simulink library "librarySimulink"  (R2020b)
settings: Solver=VariableStepAuto  StartTime=0.0  StopTime=10.0  RelTol=1e-3
values from neighbouring files (symbols this model uses):
  MU = 398600    [linearControlTuning.m]
  n = sqrt(MU/a^3)    [linearControlTuning.m]
undefined symbols (not defined in the file or in its folder): A0, areaValues, gravityGradient, MAGNETIC_FIELD_INCLINATION, magneticTorque, N_EARTH, normalVects, nSurfaces, OBLIQUITY, orbit, positions, R_EARTH, rhoDValues, rhoSValues, spacecraft, SRP
libraries: $bdroot x34
settings Model: Creator=pacif  LastModifiedBy=pacif

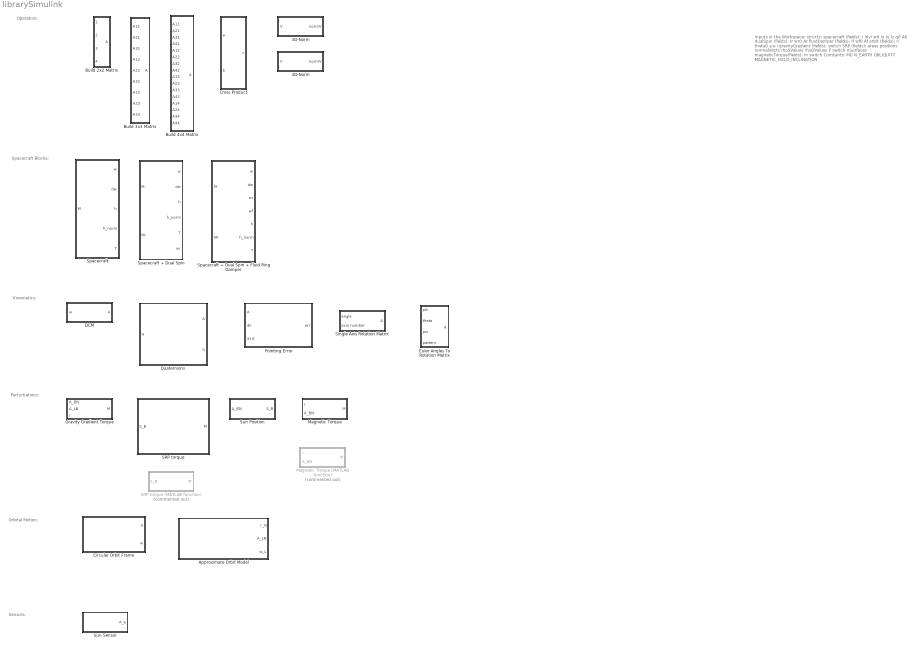
== system librarySimulink ==
  note: Operators:
  note: Inputs in the Workspace:
      |
      | structs:
      | spacecraft (fields):
      | I
      | invI
      | w0
      | Ix
      | Iy
      | Iz
      | q0
      | A0
      |
      | dualSpin (fields):
      | Ir
      | wr0
      | Ar
      | fluidDamper (fields):
      | If
      | wf0
      | Af
      | orbit (fields):
      | n
      | theta0
      | a
      | e
      | i
      | gravityGradient (fields):
      | switch
      | SRP (fields):
      | areas
      | positions
      | normalVects
      | rhoSValues
      | rhoDValues
      | P
      | switch
      | nSurfaces
      | magneticTorque(fields):
      | m
      | switch
      |
      | Constants:
      | MU
      | N_EARTH
      | OBLIQUITY
      | MAGNETIC_FIELD_INCLINATION
  note: Spacecraft Blocks:
  note: Kinematics:
  note: Perturbations:
  note: Orbital Motion:
  note: Sensors:
  3D-Norm : Subsystem
  4D-Norm : Subsystem
  Approximate Orbit Model : Subsystem
  Build 2x2 Matrix : Subsystem
  Build 3x3 Matrix : Subsystem
  Build 4x4 Matrix : Subsystem
  "Circular Orbit Frame " : Subsystem
  Cross Product : Subsystem
  DCM : Subsystem
  Euler Angles To Rotation Matrix : Subsystem
  Gravity Gradient Torque : Subsystem
  Magnetic Torque : Subsystem
  Magnetic Torque (MATLAB function) : Subsystem  Commented=on
  Pointing Error : Subsystem
  "Quaternions " : Subsystem
  SRP torque : Subsystem
  SRP torque (MATLAB function) : Subsystem  Commented=on
  Single Axis Rotation Matrix : Subsystem
  "Spacecraft " : Subsystem
  Spacecraft + Dual Spin : Subsystem  AncestorBlock=my_SADC_library/Spacecraft
  Spacecraft + Dual Spin + Fluid Ring Damper : Subsystem  AncestorBlock=my_SADC_library/Spacecraft
  "Sun Position " : Subsystem
  Sun Sensor : Subsystem

== system librarySimulink/3D-Norm ==
  V : Inport
  Add : Sum  Inputs=+++
  Demux : Demux  Outputs=3
  Square : Math  Operator=square  SaturateOnIntegerOverflow=on
  Square Root : Sqrt  SaturateOnIntegerOverflow=on
  Square1 : Math  Operator=square  SaturateOnIntegerOverflow=on
  Square2 : Math  Operator=square  SaturateOnIntegerOverflow=on
  normV : Outport
  wires:
  V/1 -> Demux/1
  Demux/3 -> Square2/1
  Demux/2 -> Square1/1
  Demux/1 -> Square/1
  Square/1 -> Add/1
  Square1/1 -> Add/2
  Square2/1 -> Add/3
  Add/1 -> Square Root/1
  Square Root/1 -> normV/1

== system librarySimulink/4D-Norm ==
  V : Inport
  Add : Sum  Inputs=++++
  Demux : Demux
  Square{,1..3} (4 alike) : Math  Operator=square  SaturateOnIntegerOverflow=on
  Square Root : Sqrt  SaturateOnIntegerOverflow=on
  normV : Outport
  wires:
  Square1/1 -> Add/2
  Demux/2 -> Square1/1
  V/1 -> Demux/1
  Demux/1 -> Square/1
  Square Root/1 -> normV/1
  Square2/1 -> Add/3
  Square/1 -> Add/1
  Demux/3 -> Square2/1
  Add/1 -> Square Root/1
  Demux/4 -> Square3/1
  Square3/1 -> Add/4

== system librarySimulink/Approximate Orbit Model ==
  Constant : Constant  Value=0
  Integrator : Integrator  InitialCondition=orbit.theta0
  Mux : Mux  Inputs=3
  Subsystem : Subsystem
  Subsystem1 : Subsystem
  Subsystem2 : Subsystem
  r_N : Outport
  A_LN : Outport  Port=2
  w_L : Outport  Port=3
  wires:
  Integrator/1 -> Subsystem2/1(theta), Subsystem1/1(theta), Subsystem/1(theta)
  Subsystem2/1(r_N) -> r_N/1
  Subsystem/1(theta_dot) -> Mux/3, Integrator/1
  Subsystem1/1(A_LN) -> A_LN/1
  Mux/1 -> w_L/1
  Constant/1 -> Mux/2, Mux/1

== system librarySimulink/Build 2x2 Matrix ==
  A11 : Inport
  A21 : Inport  Port=2
  A12 : Inport  Port=3
  A22 : Inport  Port=4
  Mux : Mux  Inputs=2
  Mux1 : Mux  Inputs=2
  Vector Concatenate : Concatenate  Mode=Multidimensional array  ConcatenateDimension=2
  A : Outport
  wires:
  Mux/1 -> Vector Concatenate/1
  Mux1/1 -> Vector Concatenate/2
  Vector Concatenate/1 -> A/1
  A11/1 -> Mux/1
  A22/1 -> Mux1/2
  A21/1 -> Mux/2
  A12/1 -> Mux1/1

== system librarySimulink/Build 3x3 Matrix ==
  A11 : Inport
  A21 : Inport  Port=2
  A31 : Inport  Port=3
  A12 : Inport  Port=4
  A22 : Inport  Port=5
  A32 : Inport  Port=6
  "A13 " : Inport  Port=7
  A23 : Inport  Port=8
  A33 : Inport  Port=9
  Mux : Mux  Inputs=3
  Mux1 : Mux  Inputs=3
  Mux2 : Mux  Inputs=3
  Vector Concatenate : Concatenate  NumInputs=3  Mode=Multidimensional array  ConcatenateDimension=2
  A : Outport
  wires:
  A11/1 -> Mux/1
  A21/1 -> Mux/2
  A31/1 -> Mux/3
  A12/1 -> Mux1/1
  A22/1 -> Mux1/2
  A32/1 -> Mux1/3
  "A13 "/1 -> Mux2/1
  A23/1 -> Mux2/2
  A33/1 -> Mux2/3
  Mux/1 -> Vector Concatenate/1
  Mux1/1 -> Vector Concatenate/2
  Mux2/1 -> Vector Concatenate/3
  Vector Concatenate/1 -> A/1

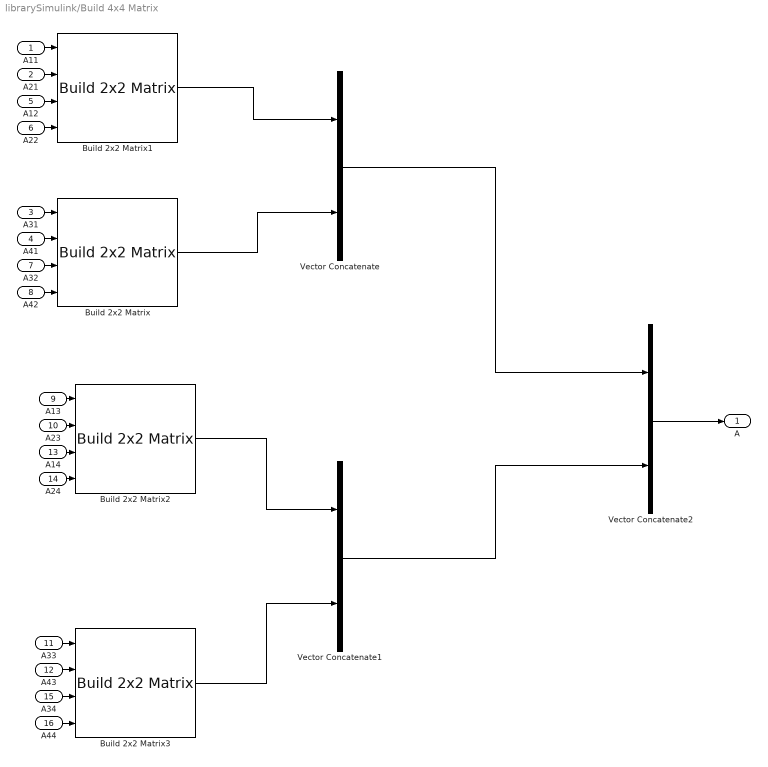
== system librarySimulink/Build 4x4 Matrix ==
  A11 : Inport
  A21 : Inport  Port=2
  A31 : Inport  Port=3
  A41 : Inport  Port=4
  A12 : Inport  Port=5
  A22 : Inport  Port=6
  A32 : Inport  Port=7
  A42 : Inport  Port=8
  A13 : Inport  Port=9
  A23 : Inport  Port=10
  A33 : Inport  Port=11
  A43 : Inport  Port=12
  A14 : Inport  Port=13
  A24 : Inport  Port=14
  A34 : Inport  Port=15
  A44 : Inport  Port=16
  Build 2x2 Matrix{,1..3} (4 alike) : $bdroot/Build 2x2 Matrix  SystemSampleTime=-1  VariantActivationTime=update diagram  Latency=0  AutoFrameSizeCalculation=off
  Vector Concatenate : Concatenate  Mode=Multidimensional array
  Vector Concatenate1 : Concatenate  Mode=Multidimensional array
  Vector Concatenate2 : Concatenate  Mode=Multidimensional array  ConcatenateDimension=2
  A : Outport
  wires:
  A11/1 -> Build 2x2 Matrix1/1
  A21/1 -> Build 2x2 Matrix1/2
  A12/1 -> Build 2x2 Matrix1/3
  A22/1 -> Build 2x2 Matrix1/4
  A13/1 -> Build 2x2 Matrix2/1
  A23/1 -> Build 2x2 Matrix2/2
  A14/1 -> Build 2x2 Matrix2/3
  A24/1 -> Build 2x2 Matrix2/4
  A31/1 -> Build 2x2 Matrix/1
  A41/1 -> Build 2x2 Matrix/2
  A32/1 -> Build 2x2 Matrix/3
  A42/1 -> Build 2x2 Matrix/4
  A33/1 -> Build 2x2 Matrix3/1
  A43/1 -> Build 2x2 Matrix3/2
  A34/1 -> Build 2x2 Matrix3/3
  A44/1 -> Build 2x2 Matrix3/4
  Build 2x2 Matrix1/1 -> Vector Concatenate/1
  Build 2x2 Matrix/1 -> Vector Concatenate/2
  Vector Concatenate/1 -> Vector Concatenate2/1
  Vector Concatenate1/1 -> Vector Concatenate2/2
  Vector Concatenate2/1 -> A/1
  Build 2x2 Matrix3/1 -> Vector Concatenate1/2
  Build 2x2 Matrix2/1 -> Vector Concatenate1/1

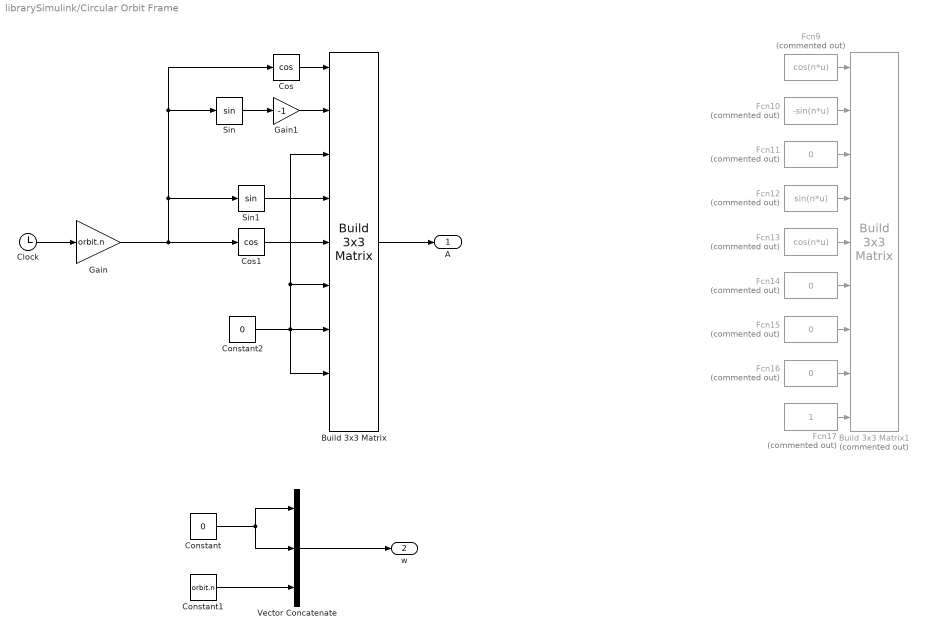
== system librarySimulink/Circular Orbit Frame  ==
  Build 3x3 Matrix : $bdroot/Build 3x3 Matrix  SystemSampleTime=-1  VariantActivationTime=update diagram  Latency=0  AutoFrameSizeCalculation=off
  Build 3x3 Matrix1 : $bdroot/Build 3x3 Matrix  Commented=on  SystemSampleTime=-1  VariantActivationTime=update diagram  Latency=0  AutoFrameSizeCalculation=off
  Clock : Clock
  Constant : Constant  Value=0
  Constant1 : Constant  Value=orbit.n
  Constant2 : Constant  Value=0
  Cos : Trigonometry  Operator=cos
  Cos1 : Trigonometry  Operator=cos
  Fcn10 : Fcn  Commented=on  Expr=-sin(n*u)
  Fcn{11,14..16} (4 alike) : Fcn  Commented=on  Expr=0
  Fcn12 : Fcn  Commented=on  Expr=sin(n*u)
  Fcn13 : Fcn  Commented=on  Expr=cos(n*u)
  Fcn17 : Fcn  Commented=on  Expr=1
  Fcn9 : Fcn  Commented=on  Expr=cos(n*u)
  Gain : Gain  Gain=orbit.n
  Gain1 : Gain  Gain=-1
  Sin : Trigonometry
  Sin1 : Trigonometry
  Vector Concatenate : Concatenate  NumInputs=3
  A : Outport
  w : Outport  Port=2
  wires:
  Cos/1 -> Build 3x3 Matrix/1
  Gain1/1 -> Build 3x3 Matrix/2
  Constant2/1 -> Build 3x3 Matrix/8, Build 3x3 Matrix/6, Build 3x3 Matrix/3, Build 3x3 Matrix/7
  Sin1/1 -> Build 3x3 Matrix/4
  Cos1/1 -> Build 3x3 Matrix/5
  ? -> Build 3x3 Matrix/9
  Constant1/1 -> Vector Concatenate/3
  Constant/1 -> Vector Concatenate/2, Vector Concatenate/1
  Vector Concatenate/1 -> w/1
  Build 3x3 Matrix/1 -> A/1
  Fcn10/1 -> Build 3x3 Matrix1/2
  Fcn14/1 -> Build 3x3 Matrix1/6
  Fcn12/1 -> Build 3x3 Matrix1/4
  Fcn17/1 -> Build 3x3 Matrix1/9
  Fcn13/1 -> Build 3x3 Matrix1/5
  Fcn16/1 -> Build 3x3 Matrix1/8
  Fcn9/1 -> Build 3x3 Matrix1/1
  Fcn15/1 -> Build 3x3 Matrix1/7
  Fcn11/1 -> Build 3x3 Matrix1/3
  Clock/1 -> Gain/1
  Sin/1 -> Gain1/1
  Gain/1 -> Cos1/1, Sin/1, Cos/1, Sin1/1

== system librarySimulink/Cross Product ==
  a : Inport
  b : Inport  Port=2
  Add : Sum  Inputs=+-
  Add1 : Sum  Inputs=+-
  Add2 : Sum  Inputs=+-
  Demux : Demux  Outputs=3
  Demux1 : Demux  Outputs=3
  Product{,1..5} (6 alike) : Product
  Vector Concatenate : Concatenate  NumInputs=3
  c : Outport
  wires:
  a/1 -> Demux/1
  Demux/2 -> Product/1, Product5/1  "Ay"
  Demux/3 -> Product1/1, Product2/1  "Az"
  b/1 -> Demux1/1
  Demux1/3 -> Product3/2, Product/2  "Bz"
  Demux1/1 -> Product5/2, Product2/2  "Bx"
  Demux1/2 -> Product1/2, Product4/2  "By"
  Vector Concatenate/1 -> c/1
  Add/1 -> Vector Concatenate/1
  Product/1 -> Add/1
  Product1/1 -> Add/2
  Add1/1 -> Vector Concatenate/2
  Add2/1 -> Vector Concatenate/3
  Product2/1 -> Add1/1
  Demux/1 -> Product4/1, Product3/1  "Ax"
  Product3/1 -> Add1/2
  Product4/1 -> Add2/1
  Product5/1 -> Add2/2

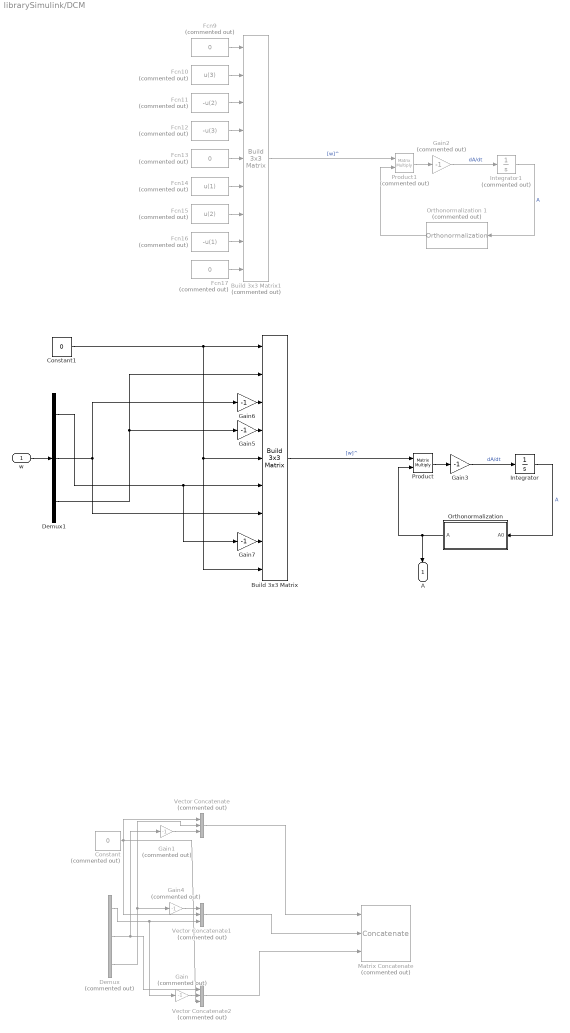
== system librarySimulink/DCM ==
  w : Inport
  Build 3x3 Matrix : $bdroot/Build 3x3 Matrix  SystemSampleTime=-1  VariantActivationTime=update diagram  Latency=0  AutoFrameSizeCalculation=off
  Build 3x3 Matrix1 : $bdroot/Build 3x3 Matrix  Commented=on  SystemSampleTime=-1  VariantActivationTime=update diagram  Latency=0  AutoFrameSizeCalculation=off
  Constant : Constant  Commented=on  Value=0
  Constant1 : Constant  Value=0
  Demux : Demux  Commented=on  Outputs=3
  Demux1 : Demux  Outputs=3
  Fcn10 : Fcn  Commented=on  Expr=u(3)
  Fcn11 : Fcn  Commented=on  Expr=-u(2)
  Fcn12 : Fcn  Commented=on  Expr=-u(3)
  Fcn13 : Fcn  Commented=on  Expr=0
  Fcn14 : Fcn  Commented=on  Expr=u(1)
  Fcn15 : Fcn  Commented=on  Expr=u(2)
  Fcn16 : Fcn  Commented=on  Expr=-u(1)
  Fcn17 : Fcn  Commented=on  Expr=0
  Fcn9 : Fcn  Commented=on  Expr=0
  Gain{,1..2,4} (4 alike) : Gain  Commented=on  Gain=-1
  Gain{3,5..7} (4 alike) : Gain  Gain=-1
  Integrator : Integrator  InitialCondition=spacecraft.A0
  Integrator1 : Integrator  Commented=on  InitialCondition=A0
  Matrix Concatenate : Concatenate  Commented=on  NumInputs=3  Mode=Multidimensional array  ConcatenateDimension=2
  "Orthonormalization " : Subsystem  AncestorBlock=my_SADC_library/DCM/Orthonormalization
  Orthonormalization 1 : $bdroot/DCM/Orthonormalization   Commented=on  SystemSampleTime=-1  VariantActivationTime=update diagram  Latency=0  AutoFrameSizeCalculation=off
  Product : Product  Multiplication=Matrix(*)
  Product1 : Product  Commented=on  Multiplication=Matrix(*)
  Vector Concatenate : Concatenate  Commented=on  NumInputs=3
  Vector Concatenate1 : Concatenate  Commented=on  NumInputs=3
  Vector Concatenate2 : Concatenate  Commented=on  NumInputs=3
  A : Outport
  wires:
  Product/1 -> Gain3/1
  Integrator/1 -> "Orthonormalization "/1(A0)  "A"
  Gain3/1 -> Integrator/1  "dA/dt"
  "Orthonormalization "/1(A) -> Product/2, A/1
  Gain1/1 -> Vector Concatenate/3
  Vector Concatenate/1 -> Matrix Concatenate/1
  Demux/3 -> Gain4/1, Vector Concatenate/2
  Gain4/1 -> Vector Concatenate1/1
  Gain/1 -> Vector Concatenate2/2
  Vector Concatenate1/1 -> Matrix Concatenate/2
  Demux/2 -> Vector Concatenate2/1, Gain1/1
  Demux/1 -> Gain/1, Vector Concatenate1/3
  Constant/1 -> Vector Concatenate2/3, Vector Concatenate1/2, Vector Concatenate/1
  Vector Concatenate2/1 -> Matrix Concatenate/3
  Build 3x3 Matrix/1 -> Product/1  "[w]^"
  Constant1/1 -> Build 3x3 Matrix/5, Build 3x3 Matrix/9, Build 3x3 Matrix/1
  Fcn11/1 -> Build 3x3 Matrix1/3
  Fcn17/1 -> Build 3x3 Matrix1/9
  Fcn13/1 -> Build 3x3 Matrix1/5
  Fcn16/1 -> Build 3x3 Matrix1/8
  Fcn15/1 -> Build 3x3 Matrix1/7
  Fcn14/1 -> Build 3x3 Matrix1/6
  Build 3x3 Matrix1/1 -> Product1/1  "[w]^"
  Fcn10/1 -> Build 3x3 Matrix1/2
  Fcn9/1 -> Build 3x3 Matrix1/1
  Fcn12/1 -> Build 3x3 Matrix1/4
  Integrator1/1 -> Orthonormalization 1/1  "A"
  Gain2/1 -> Integrator1/1  "dA/dt"
  Orthonormalization 1/1 -> Product1/2
  Product1/1 -> Gain2/1
  w/1 -> Demux1/1
  Gain6/1 -> Build 3x3 Matrix/3
  Gain5/1 -> Build 3x3 Matrix/4
  Gain7/1 -> Build 3x3 Matrix/8
  Demux1/3 -> Gain5/1, Build 3x3 Matrix/2
  Demux1/2 -> Build 3x3 Matrix/7, Gain6/1
  Demux1/1 -> Gain7/1, Build 3x3 Matrix/6

== system librarySimulink/Euler Angles To Rotation Matrix ==
  phi : Inport
  theta : Inport  Port=2
  psi : Inport  Port=3
  pattern : Inport  Port=4
  Demux : Demux  Outputs=3
  Product : Product  Inputs=3  Multiplication=Matrix(*)
  Single Axis Rotation Matrix : $bdroot/Single Axis Rotation Matrix  SystemSampleTime=-1  VariantActivationTime=update diagram  Latency=0  AutoFrameSizeCalculation=off
  Single Axis Rotation Matrix1 : $bdroot/Single Axis Rotation Matrix  SystemSampleTime=-1  VariantActivationTime=update diagram  Latency=0  AutoFrameSizeCalculation=off
  Single Axis Rotation Matrix2 : $bdroot/Single Axis Rotation Matrix  SystemSampleTime=-1  VariantActivationTime=update diagram  Latency=0  AutoFrameSizeCalculation=off
  A : Outport
  wires:
  pattern/1 -> Demux/1
  Demux/1 -> Single Axis Rotation Matrix/2
  Demux/2 -> Single Axis Rotation Matrix1/2
  Demux/3 -> Single Axis Rotation Matrix2/2
  phi/1 -> Single Axis Rotation Matrix/1
  theta/1 -> Single Axis Rotation Matrix1/1
  psi/1 -> Single Axis Rotation Matrix2/1
  Single Axis Rotation Matrix2/1 -> Product/1
  Single Axis Rotation Matrix1/1 -> Product/2
  Single Axis Rotation Matrix/1 -> Product/3
  Product/1 -> A/1

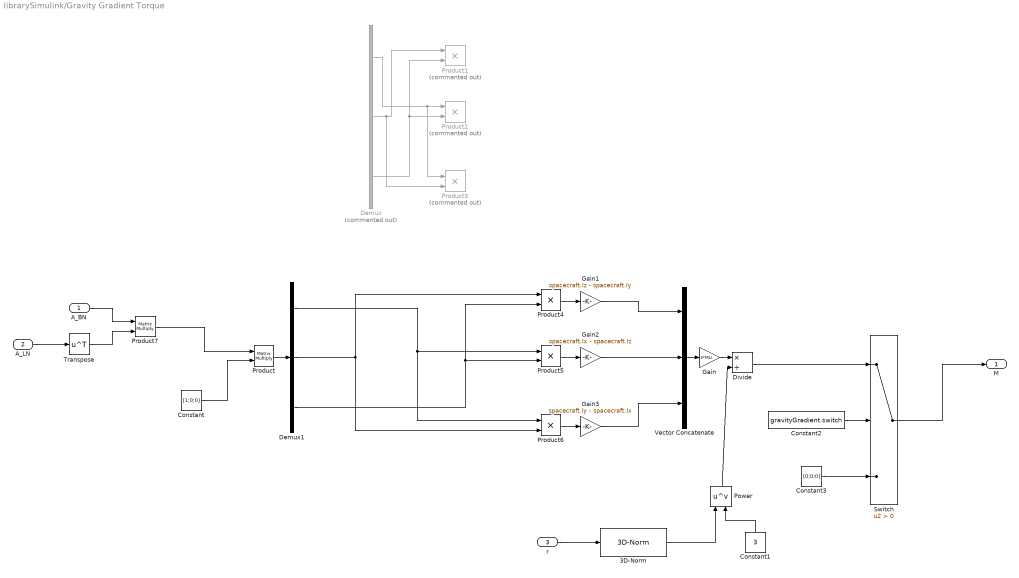
== system librarySimulink/Gravity Gradient Torque ==
  A_BN : Inport
  A_LN : Inport  Port=2
  r : Inport  Port=3
  3D-Norm : $bdroot/3D-Norm  SystemSampleTime=-1  VariantActivationTime=update diagram  Latency=0  AutoFrameSizeCalculation=off
  Constant : Constant  Value=[1;0;0]  VectorParams1D=off
  Constant1 : Constant  Value=3
  Constant2 : Constant  Value=gravityGradient.switch
  Constant3 : Constant  Value=[0;0;0]
  Demux : Demux  Commented=on  Outputs=3
  Demux1 : Demux  Outputs=3
  Divide : Product  Inputs=*/
  Gain : Gain  Gain=3*MU
  Gain1 : Gain  Gain=spacecraft.Iz - spacecraft.Iy
  Gain2 : Gain  Gain=spacecraft.Ix - spacecraft.Iz
  Gain3 : Gain  Gain=spacecraft.Iy - spacecraft.Ix
  Power : Math  Operator=pow  SaturateOnIntegerOverflow=on
  Product : Product  Multiplication=Matrix(*)
  Product1 : Product  Commented=on
  Product2 : Product  Commented=on
  Product3 : Product  Commented=on
  Product4 : Product
  Product5 : Product
  Product6 : Product
  Product7 : Product  Multiplication=Matrix(*)
  Switch : Switch  Criteria=u2 > Threshold
  Transpose : Math  Operator=transpose  SaturateOnIntegerOverflow=on
  Vector Concatenate : Concatenate  NumInputs=3
  M : Outport
  wires:
  Demux/3 -> Product2/2, Product1/2
  Demux/2 -> Product3/2, Product1/1
  Demux/1 -> Product3/1, Product2/1
  Constant/1 -> Product/2
  Gain3/1 -> Vector Concatenate/3
  Gain1/1 -> Vector Concatenate/1
  Gain2/1 -> Vector Concatenate/2
  Vector Concatenate/1 -> Gain/1
  Constant1/1 -> Power/2
  Power/1 -> Divide/2
  Gain/1 -> Divide/1
  Product/1 -> Demux1/1
  Product4/1 -> Gain1/1
  Product5/1 -> Gain2/1
  Product6/1 -> Gain3/1
  Demux1/1 -> Product6/1, Product5/1
  Demux1/2 -> Product6/2, Product4/1
  Demux1/3 -> Product5/2, Product4/2
  Switch/1 -> M/1
  Divide/1 -> Switch/1
  Constant2/1 -> Switch/2
  Constant3/1 -> Switch/3
  r/1 -> 3D-Norm/1
  3D-Norm/1 -> Power/1
  A_LN/1 -> Transpose/1
  Product7/1 -> Product/1
  A_BN/1 -> Product7/1
  Transpose/1 -> Product7/2

== system librarySimulink/Magnetic Torque ==
  r : Inport
  A_BN : Inport  Port=2
  Constant2 : Constant  Value=magneticTorque.switch
  Constant3 : Constant  Value=[0;0;0]
  Cross Product : $bdroot/Cross Product  SystemSampleTime=-1  VariantActivationTime=update diagram  Latency=0  AutoFrameSizeCalculation=off
  Product : Product  Multiplication=Matrix(*)
  Subsystem : Subsystem
  Switch : Switch  Criteria=u2 > Threshold
  m : Constant  Value=magneticTorque.m
  M : Outport
  wires:
  r/1 -> Subsystem/1(r)
  A_BN/1 -> Product/1
  Subsystem/1(b_N) -> Product/2
  m/1 -> Cross Product/1
  Product/1 -> Cross Product/2
  Constant3/1 -> Switch/3
  Constant2/1 -> Switch/2
  Cross Product/1 -> Switch/1
  Switch/1 -> M/1

== system librarySimulink/Magnetic Torque (MATLAB function) ==
  r : Inport
  A_BN : Inport  Port=2
  Clock : Clock
  MATLAB Function : MATLAB Function  TreatAsAtomicUnit=on
  m : Constant  Value=magneticTorque.m
  M : Outport
  wires:
  m/1 -> MATLAB Function/4(m)
  A_BN/1 -> MATLAB Function/3(A_BN)
  r/1 -> MATLAB Function/2(r)
  Clock/1 -> MATLAB Function/1(t)
  MATLAB Function/1(M) -> M/1

== system librarySimulink/Pointing Error ==
  A : Inport
  dir : Inport  Port=2
  axis : Inport  Port=3
  Acos : Trigonometry  Operator=acos
  Dot Product : DotProduct  InputSameDT=on  OutDataTypeStr=Inherit: Inherit via internal rule
  Product : Product  Multiplication=Matrix(*)
  err : Outport
  wires:
  A/1 -> Product/1
  axis/1 -> Dot Product/2
  Product/1 -> Dot Product/1
  Dot Product/1 -> Acos/1
  Acos/1 -> err/1
  dir/1 -> Product/2

== system librarySimulink/Quaternions  ==
  w : Inport
  Gain : Gain  Gain=0.5
  Integrator : Integrator  InitialCondition=spacecraft.q0
  M1 : Subsystem
  M2 : Subsystem
  "Normalization " : Subsystem
  Product : Product  Multiplication=Matrix(*)
  A : Outport
  q : Outport  Port=2
  wires:
  w/1 -> M1/1(w)
  M1/1(M1) -> Gain/1
  Gain/1 -> Product/1
  Product/1 -> Integrator/1  "q_dot"
  Integrator/1 -> "Normalization "/1("q ")  "q"
  M2/1("M2 ") -> A/1
  "Normalization "/1(qNormalized) -> M2/1(q), q/1, Product/2

== system librarySimulink/SRP torque ==
  S_B : Inport
  Constant2 : Constant  Value=SRP.switch
  Constant3 : Constant  Value=[0;0;0]
  For Iterator Subsystem : Subsystem  TreatAsAtomicUnit=on
  Switch : Switch  Criteria=u2 > Threshold
  M : Outport
  wires:
  S_B/1 -> For Iterator Subsystem/1(S_B)
  Constant3/1 -> Switch/3
  Constant2/1 -> Switch/2
  Switch/1 -> M/1
  For Iterator Subsystem/1(T) -> Switch/1

== system librarySimulink/SRP torque (MATLAB function) ==
  S_B : Inport
  Constant : Constant  Value=areaValues  VectorParams1D=off
  Constant1 : Constant  Value=positions  VectorParams1D=off
  Constant2 : Constant  Value=normalVects  VectorParams1D=off
  Constant3 : Constant  Value=rhoSValues  VectorParams1D=off
  Constant4 : Constant  Value=rhoDValues  VectorParams1D=off
  MATLAB Function : MATLAB Function  TreatAsAtomicUnit=on
  M : Outport
  wires:
  MATLAB Function/1(M) -> M/1
  S_B/1 -> MATLAB Function/1(S_B)
  Constant/1 -> MATLAB Function/2(areaValues)
  Constant1/1 -> MATLAB Function/3(positions)
  Constant2/1 -> MATLAB Function/4(normalVects)
  Constant3/1 -> MATLAB Function/5(rhoSValues)
  Constant4/1 -> MATLAB Function/6(rhoDValues)

== system librarySimulink/Single Axis Rotation Matrix ==
  angle : Inport
  axis number : Inport  Port=2
  If : If  IfExpression=u1 == 1  ElseIfExpressions=u1 == 2, u1 == 3  ShowElse=off
  If Action Subsystem : Subsystem  TreatAsAtomicUnit=on
  If Action Subsystem1 : Subsystem  AncestorBlock=mySADCLibrary/Subsystem/If Action Subsystem  TreatAsAtomicUnit=on
  If Action Subsystem2 : Subsystem  AncestorBlock=mySADCLibrary/Subsystem/If Action Subsystem  TreatAsAtomicUnit=on
  Merge : Merge  Inputs=3
  A : Outport
  wires:
  axis number/1 -> If/1
  If/1 -> If Action Subsystem/Action
  If/2 -> If Action Subsystem1/Action
  If/3 -> If Action Subsystem2/Action
  angle/1 -> If Action Subsystem/1(angle), If Action Subsystem1/1(angle), If Action Subsystem2/1(angle)
  Merge/1 -> A/1
  If Action Subsystem/1(A) -> Merge/1
  If Action Subsystem1/1(A) -> Merge/2
  If Action Subsystem2/1(A) -> Merge/3

== system librarySimulink/Spacecraft  ==
  M : Inport
  3D-Norm : $bdroot/3D-Norm  SystemSampleTime=-1  VariantActivationTime=update diagram  Latency=0  AutoFrameSizeCalculation=off
  Add : Sum
  Cross Product : $bdroot/Cross Product  SystemSampleTime=-1  VariantActivationTime=update diagram  Latency=0  AutoFrameSizeCalculation=off
  Dot Product : DotProduct  InputSameDT=on  OutDataTypeStr=Inherit: Inherit via internal rule
  Gain : Gain  Gain=spacecraft.invI  Multiplication=Matrix(K*u) (u vector)
  Gain1 : Gain  Gain=1/2*spacecraft.I  Multiplication=Matrix(K*u) (u vector)
  Gain2 : Gain  Gain=spacecraft.I  Multiplication=Matrix(K*u) (u vector)
  Integrator : Integrator  InitialCondition=spacecraft.w0
  w : Outport
  dw : Outport  Port=2
  h : Outport  Port=3
  "h_norm " : Outport  Port=4
  T : Outport  Port=5
  wires:
  Add/1 -> Gain/1
  Integrator/1 -> Cross Product/2, Gain2/1, Dot Product/2, Gain1/1, w/1  "w"
  Gain/1 -> Integrator/1, dw/1  "dw"
  Gain2/1 -> Cross Product/1, 3D-Norm/1, h/1  "I*w"
  M/1 -> Add/1
  Cross Product/1 -> Add/2  "I*w x w = -w x I*w"
  Gain1/1 -> Dot Product/1  "I*w"
  Dot Product/1 -> T/1
  3D-Norm/1 -> "h_norm "/1

== system librarySimulink/Spacecraft + Dual Spin ==
  M : Inport
  Mr : Inport  Port=2
  3D-Norm : $bdroot/3D-Norm  SystemSampleTime=-1  VariantActivationTime=update diagram  Latency=0  AutoFrameSizeCalculation=off
  Dual Spin : Subsystem
  Euler Equations : Subsystem
  w : Outport
  dw : Outport  Port=2
  h : Outport  Port=3
  "h_norm " : Outport  Port=4
  T : Outport  Port=5
  wr : Outport  Port=6
  wires:
  Dual Spin/1(wr) -> Euler Equations/2(wr), wr/1
  Euler Equations/1(w) -> w/1
  Euler Equations/2(dw) -> dw/1
  M/1 -> Euler Equations/1(M)
  Dual Spin/2(wr_dot) -> Euler Equations/3("wr_dot ")
  Mr/1 -> Dual Spin/1(Mr)
  Euler Equations/3(h) -> 3D-Norm/1, h/1
  Euler Equations/4(T) -> T/1
  3D-Norm/1 -> "h_norm "/1

== system librarySimulink/Spacecraft + Dual Spin + Fluid Ring Damper ==
  M : Inport
  Mr : Inport  Port=2
  3D-Norm : $bdroot/3D-Norm  SystemSampleTime=-1  VariantActivationTime=update diagram  Latency=0  AutoFrameSizeCalculation=off
  Dual Spin : $bdroot/Spacecraft + Dual Spin/Dual Spin  SystemSampleTime=-1  VariantActivationTime=update diagram  Latency=0  AutoFrameSizeCalculation=off
  Euler Equations : Subsystem  AncestorBlock=my_SADC_library/Spacecraft + Dual Spin/Euler Equations
  Fluid Ring Damper : Subsystem
  w : Outport
  dw : Outport  Port=2
  "wr " : Outport  Port=3
  wf : Outport  Port=4
  h : Outport  Port=5
  h_norm : Outport  Port=6
  T : Outport  Port=7
  wires:
  Mr/1 -> Dual Spin/1
  Euler Equations/2(dw) -> dw/1
  Euler Equations/1(w) -> w/1, Fluid Ring Damper/1(w)
  Dual Spin/2 -> Euler Equations/3("wr_dot ")
  Dual Spin/1 -> Euler Equations/2(wr), "wr "/1
  M/1 -> Euler Equations/1(M)
  Fluid Ring Damper/1(wf) -> Euler Equations/4(wf), wf/1
  Fluid Ring Damper/2(wf_dot) -> Euler Equations/5(wf_dot)
  Euler Equations/3(h) -> 3D-Norm/1, h/1
  Euler Equations/4(T) -> T/1
  3D-Norm/1 -> h_norm/1

== system librarySimulink/Sun Position  ==
  A_BN : Inport
  Clock : Clock
  Cos : Trigonometry  Operator=cos
  Gain1 : Gain  Gain=N_EARTH
  Gain2 : Gain  Gain=cos(OBLIQUITY)
  Gain3 : Gain  Gain=sin(OBLIQUITY)
  Mux : Mux  Inputs=3
  Product : Product  Multiplication=Matrix(*)
  Sin : Trigonometry
  Sin1 : Trigonometry
  S_B : Outport
  wires:
  Clock/1 -> Gain1/1
  Mux/1 -> Product/2  "S_N"
  Gain2/1 -> Mux/2
  Gain3/1 -> Mux/3
  Cos/1 -> Mux/1
  Sin1/1 -> Gain3/1
  Sin/1 -> Gain2/1
  Gain1/1 -> Sin/1, Sin1/1, Cos/1
  A_BN/1 -> Product/1
  Product/1 -> S_B/1

== system librarySimulink/Sun Sensor ==
  Constant : Constant  Value=[1;2;3]
  Euler Angles To Rotation Matrix : $bdroot/Euler Angles To Rotation Matrix  SystemSampleTime=-1  VariantActivationTime=update diagram  Latency=0  AutoFrameSizeCalculation=off
  phi : RandomNumber  Variance=1/8  SampleTime=0.1
  psi : RandomNumber  Variance=1/8  SampleTime=0.1
  theta : RandomNumber  Variance=1/8  SampleTime=0.1
  A_e : Outport
  wires:
  theta/1 -> Euler Angles To Rotation Matrix/2
  phi/1 -> Euler Angles To Rotation Matrix/1
  psi/1 -> Euler Angles To Rotation Matrix/3
  Constant/1 -> Euler Angles To Rotation Matrix/4
  Euler Angles To Rotation Matrix/1 -> A_e/1

== system librarySimulink/Approximate Orbit Model/Subsystem ==
  theta : Inport
  Add : Sum
  Constant : Constant
  Cos : Trigonometry  Operator=cos
  Gain : Gain  Gain=orbit.e
  Gain1 : Gain  Gain=orbit.n/(1-orbit.e^2)^(3/2)
  Square : Math  Operator=square  SaturateOnIntegerOverflow=on
  theta_dot : Outport
  wires:
  theta/1 -> Cos/1
  Cos/1 -> Gain/1
  Gain/1 -> Add/1
  Constant/1 -> Add/2
  Add/1 -> Square/1
  Square/1 -> Gain1/1
  Gain1/1 -> theta_dot/1

== system librarySimulink/Approximate Orbit Model/Subsystem1 ==
  theta : Inport
  Build 3x3 Matrix : $bdroot/Build 3x3 Matrix  SystemSampleTime=-1  VariantActivationTime=update diagram  Latency=0  AutoFrameSizeCalculation=off
  Constant : Constant  Value=0
  Constant1 : Constant
  Cos1 : Trigonometry  Operator=cos
  Cos2 : Trigonometry  Operator=cos
  Gain : Gain  Gain=-1
  Gain1 : Gain  Gain=[1 0 0; 0 cos(orbit.i) sin(orbit.i); 0 -sin(orbit.i) cos(orbit.i)]  Multiplication=Matrix(u*K)
  Sin : Trigonometry
  Sin1 : Trigonometry
  A_LN : Outport
  wires:
  Cos1/1 -> Build 3x3 Matrix/1
  theta/1 -> Cos2/1, Sin1/1, Cos1/1, Sin/1
  Sin/1 -> Gain/1
  Gain/1 -> Build 3x3 Matrix/2
  Sin1/1 -> Build 3x3 Matrix/4
  Cos2/1 -> Build 3x3 Matrix/5
  Constant/1 -> Build 3x3 Matrix/8, Build 3x3 Matrix/6, Build 3x3 Matrix/3, Build 3x3 Matrix/7
  Constant1/1 -> Build 3x3 Matrix/9
  Build 3x3 Matrix/1 -> Gain1/1
  Gain1/1 -> A_LN/1

== system librarySimulink/Approximate Orbit Model/Subsystem2 ==
  theta : Inport
  Add : Sum
  Constant : Constant
  Constant1 : Constant  Value=orbit.a*(1-orbit.e^2)
  Cos : Trigonometry  Operator=cos
  Cos1 : Trigonometry  Operator=cos
  Divide : Product  Inputs=/*
  Gain : Gain  Gain=cos(orbit.i)
  Gain1 : Gain  Gain=sin(orbit.i)
  Gain3 : Gain  Gain=orbit.e
  Mux : Mux  Inputs=3
  Product : Product
  Sin : Trigonometry
  Sin1 : Trigonometry
  r_N : Outport
  wires:
  Cos/1 -> Mux/1
  theta/1 -> Cos1/1, Sin1/1, Cos/1, Sin/1
  Gain/1 -> Mux/2
  Gain1/1 -> Mux/3
  Sin/1 -> Gain/1
  Sin1/1 -> Gain1/1
  Cos1/1 -> Gain3/1
  Gain3/1 -> Add/1
  Constant/1 -> Add/2
  Add/1 -> Divide/1
  Constant1/1 -> Divide/2
  Divide/1 -> Product/2
  Mux/1 -> Product/1
  Product/1 -> r_N/1

== system librarySimulink/DCM/Orthonormalization  ==
  A0 : Inport
  Add : Sum  Inputs=+-
  Gain : Gain  Gain=1.5
  Gain1 : Gain  Gain=0.5
  Product : Product  Inputs=3  Multiplication=Matrix(*)
  Transpose : Math  Operator=transpose  SaturateOnIntegerOverflow=on
  A : Outport
  wires:
  A0/1 -> Product/3, Transpose/1, Product/1, Gain/1
  Add/1 -> A/1
  Transpose/1 -> Product/2
  Product/1 -> Gain1/1
  Gain1/1 -> Add/2
  Gain/1 -> Add/1

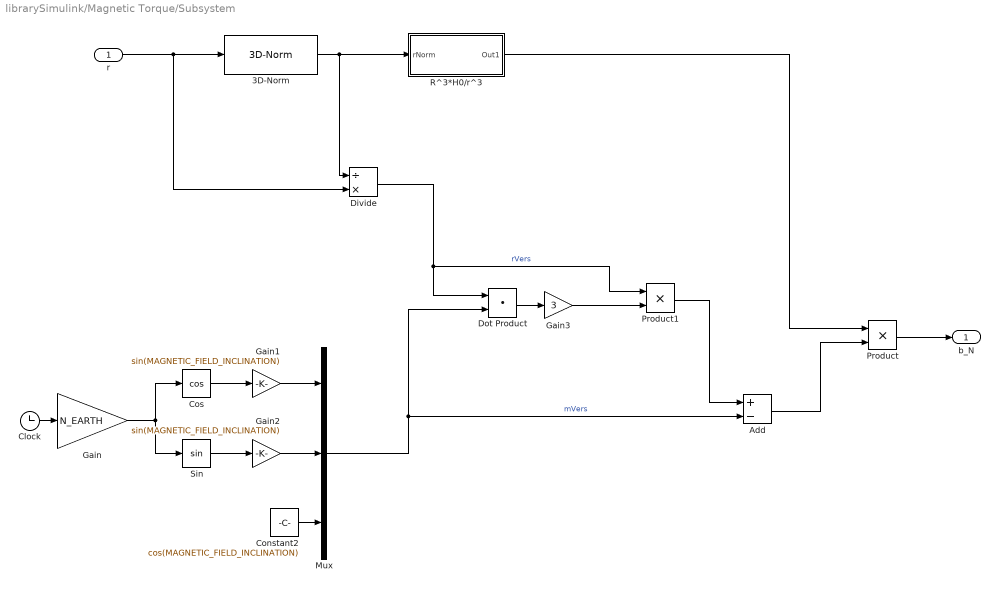
== system librarySimulink/Magnetic Torque/Subsystem ==
  r : Inport
  3D-Norm : $bdroot/3D-Norm  SystemSampleTime=-1  VariantActivationTime=update diagram  Latency=0  AutoFrameSizeCalculation=off
  Add : Sum  Inputs=+-
  Clock : Clock
  Constant2 : Constant  Value=cos(MAGNETIC_FIELD_INCLINATION)
  Cos : Trigonometry  Operator=cos
  Divide : Product  Inputs=/*
  Dot Product : DotProduct  InputSameDT=on  OutDataTypeStr=Inherit: Inherit via internal rule
  Gain : Gain  Gain=N_EARTH
  Gain1 : Gain  Gain=sin(MAGNETIC_FIELD_INCLINATION)
  Gain2 : Gain  Gain=sin(MAGNETIC_FIELD_INCLINATION)
  Gain3 : Gain  Gain=3
  Mux : Mux  Inputs=3
  Product : Product
  Product1 : Product
  R^3*H0/r^3 : Subsystem
  Sin : Trigonometry
  b_N : Outport
  wires:
  3D-Norm/1 -> Divide/1, R^3*H0/r^3/1(rNorm)
  Cos/1 -> Gain1/1
  Sin/1 -> Gain2/1
  Gain2/1 -> Mux/2
  r/1 -> Divide/2, 3D-Norm/1
  Product1/1 -> Add/1
  Gain/1 -> Sin/1, Cos/1
  Constant2/1 -> Mux/3
  Gain1/1 -> Mux/1
  Gain3/1 -> Product1/2
  Product/1 -> b_N/1
  Add/1 -> Product/2
  Clock/1 -> Gain/1
  R^3*H0/r^3/1(Out1) -> Product/1
  Dot Product/1 -> Gain3/1
  Divide/1 -> Product1/1, Dot Product/1  "rVers"
  Mux/1 -> Dot Product/2, Add/2  "mVers"

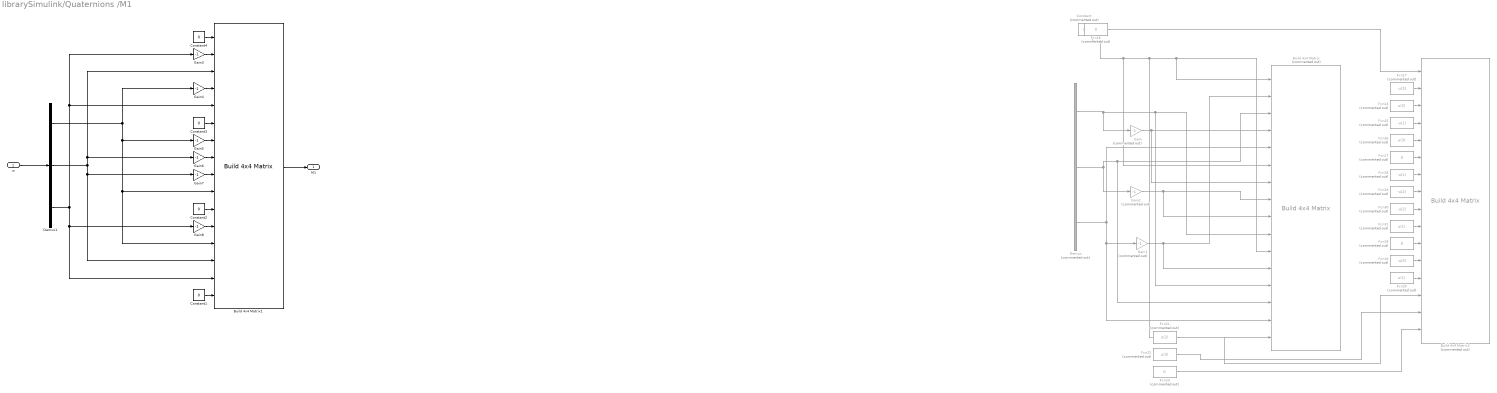
== system librarySimulink/Quaternions /M1 ==
  w : Inport
  Build 4x4 Matrix : $bdroot/Build 4x4 Matrix  Commented=on  SystemSampleTime=-1  VariantActivationTime=update diagram  Latency=0  AutoFrameSizeCalculation=off
  Build 4x4 Matrix1 : $bdroot/Build 4x4 Matrix  SystemSampleTime=-1  VariantActivationTime=update diagram  Latency=0  AutoFrameSizeCalculation=off
  Build 4x4 Matrix2 : $bdroot/Build 4x4 Matrix  Commented=on  SystemSampleTime=-1  VariantActivationTime=update diagram  Latency=0  AutoFrameSizeCalculation=off
  Constant : Constant  Commented=on  Value=0
  Constant{1..4} (4 alike) : Constant  Value=0
  Demux : Demux  Commented=on  Outputs=3
  Demux1 : Demux  Outputs=3
  Fcn{16,18,23,27} (4 alike) : Fcn  Commented=on  Expr=0
  Fcn17 : Fcn  Commented=on  Expr=-u(3)
  Fcn19 : Fcn  Commented=on  Expr=-u(3)
  Fcn20 : Fcn  Commented=on  Expr=u(1)
  Fcn21 : Fcn  Commented=on  Expr=u(2)
  Fcn22 : Fcn  Commented=on  Expr=u(3)
  Fcn24 : Fcn  Commented=on  Expr=u(2)
  Fcn25 : Fcn  Commented=on  Expr=-u(1)
  Fcn26 : Fcn  Commented=on  Expr=u(3)
  Fcn28 : Fcn  Commented=on  Expr=-u(1)
  Fcn29 : Fcn  Commented=on  Expr=-u(2)
  Fcn30 : Fcn  Commented=on  Expr=-u(2)
  Fcn31 : Fcn  Commented=on  Expr=u(1)
  Gain : Gain  Commented=on  Gain=-1
  Gain1 : Gain  Commented=on  Gain=-1
  Gain2 : Gain  Commented=on  Gain=-1
  Gain{3..8} (6 alike) : Gain  Gain=-1
  M1 : Outport
  wires:
  Demux/1 -> Build 4x4 Matrix/13, Build 4x4 Matrix/10, Gain/1
  Demux/3 -> Build 4x4 Matrix/15, Gain1/1, Build 4x4 Matrix/5
  Demux/2 -> Build 4x4 Matrix/14, Build 4x4 Matrix/3, Gain2/1
  Constant/1 -> Build 4x4 Matrix/6, Build 4x4 Matrix/16, Build 4x4 Matrix/11, Build 4x4 Matrix/1
  Gain1/1 -> Build 4x4 Matrix/12, Build 4x4 Matrix/2
  Gain/1 -> Build 4x4 Matrix/7, Build 4x4 Matrix/4
  Gain2/1 -> Build 4x4 Matrix/9, Build 4x4 Matrix/8
  Build 4x4 Matrix1/1 -> M1/1
  Constant4/1 -> Build 4x4 Matrix1/1
  Gain3/1 -> Build 4x4 Matrix1/2
  Gain4/1 -> Build 4x4 Matrix1/4
  Gain5/1 -> Build 4x4 Matrix1/7
  Gain6/1 -> Build 4x4 Matrix1/8
  Constant3/1 -> Build 4x4 Matrix1/6
  Gain7/1 -> Build 4x4 Matrix1/9
  Constant2/1 -> Build 4x4 Matrix1/11
  Gain8/1 -> Build 4x4 Matrix1/12
  Demux1/1 -> Build 4x4 Matrix1/13, Build 4x4 Matrix1/10, Gain5/1, Gain4/1
  Demux1/3 -> Build 4x4 Matrix1/15, Gain8/1, Gain3/1, Build 4x4 Matrix1/5
  Constant1/1 -> Build 4x4 Matrix1/16
  Demux1/2 -> Build 4x4 Matrix1/14, Gain7/1, Build 4x4 Matrix1/3, Gain6/1
  Fcn28/1 -> Build 4x4 Matrix2/7
  Fcn26/1 -> Build 4x4 Matrix2/5
  Fcn16/1 -> Build 4x4 Matrix2/1
  Fcn31/1 -> Build 4x4 Matrix2/10
  Fcn17/1 -> Build 4x4 Matrix2/2
  Fcn27/1 -> Build 4x4 Matrix2/6
  Fcn25/1 -> Build 4x4 Matrix2/4
  Fcn30/1 -> Build 4x4 Matrix2/9
  Fcn21/1 -> Build 4x4 Matrix2/14
  Fcn22/1 -> Build 4x4 Matrix2/15
  Fcn18/1 -> Build 4x4 Matrix2/11
  Fcn20/1 -> Build 4x4 Matrix2/13
  Fcn19/1 -> Build 4x4 Matrix2/12
  Fcn29/1 -> Build 4x4 Matrix2/8
  Fcn23/1 -> Build 4x4 Matrix2/16
  Fcn24/1 -> Build 4x4 Matrix2/3
  w/1 -> Demux1/1

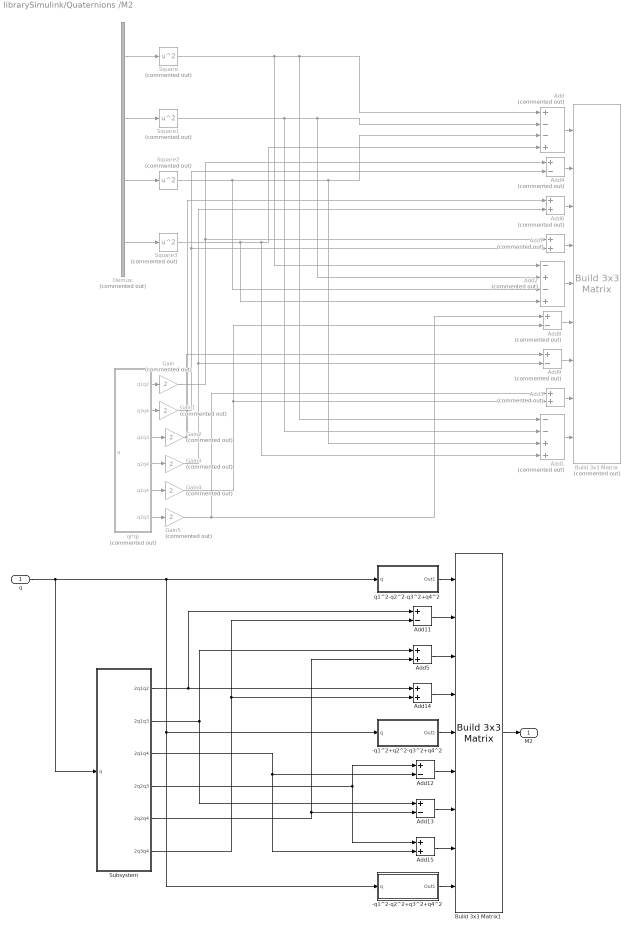
== system librarySimulink/Quaternions /M2 ==
  q : Inport
  -q1^2+q2^2-q3^2+q4^2 : Subsystem  AncestorBlock=my_SADC_library/Quaternions /M2/q1^2-q2^2-q3^2+q4^2
  -q1^2-q2^2+q3^2+q4^2 : Subsystem  AncestorBlock=my_SADC_library/Quaternions /M2/q1^2-q2^2-q3^2+q4^2
  Add : Sum  Commented=on  Inputs=+--+
  Add1 : Sum  Commented=on  Inputs=--++
  Add11 : Sum  Inputs=+-
  Add12 : Sum  Inputs=+-
  Add13 : Sum  Inputs=+-
  Add14 : Sum
  Add15 : Sum
  Add2 : Sum  Commented=on  Inputs=-+-+
  Add3 : Sum  Commented=on
  Add4 : Sum  Commented=on  Inputs=+-
  Add5 : Sum
  Add6 : Sum  Commented=on
  Add7 : Sum  Commented=on
  Add8 : Sum  Commented=on  Inputs=+-
  Add9 : Sum  Commented=on  Inputs=+-
  Build 3x3 Matrix : $bdroot/Build 3x3 Matrix  Commented=on  SystemSampleTime=-1  VariantActivationTime=update diagram  Latency=0  AutoFrameSizeCalculation=off
  Build 3x3 Matrix1 : $bdroot/Build 3x3 Matrix  SystemSampleTime=-1  VariantActivationTime=update diagram  Latency=0  AutoFrameSizeCalculation=off
  Demux : Demux  Commented=on
  Gain{,1..5} (6 alike) : Gain  Commented=on  Gain=2
  Square{,1..3} (4 alike) : Math  Commented=on  Operator=square  SaturateOnIntegerOverflow=on
  Subsystem : Subsystem
  q1^2-q2^2-q3^2+q4^2 : Subsystem
  "qi*qj " : Subsystem  Commented=on
  "M2 " : Outport
  wires:
  Demux/1 -> Square/1
  Demux/2 -> Square1/1
  Demux/3 -> Square2/1
  Demux/4 -> Square3/1
  Add/1 -> Build 3x3 Matrix/1
  Square/1 -> Add2/1, Add1/1, Add/1
  Square1/1 -> Add1/2, Add2/2, Add/2
  Square2/1 -> Add2/3, Add1/3, Add/3
  Square3/1 -> Add2/4, Add1/4, Add/4
  "qi*qj "/1(q1q2) -> Gain/1
  "qi*qj "/2(q3q4) -> Gain1/1
  "qi*qj "/3(q1q3) -> Gain2/1
  "qi*qj "/4(q2q4) -> Gain3/1
  "qi*qj "/5(q1q4) -> Gain4/1
  "qi*qj "/6(q2q3) -> Gain5/1
  Add2/1 -> Build 3x3 Matrix/5
  Add1/1 -> Build 3x3 Matrix/9
  Add4/1 -> Build 3x3 Matrix/2
  Add6/1 -> Build 3x3 Matrix/3
  Add7/1 -> Build 3x3 Matrix/4
  Add8/1 -> Build 3x3 Matrix/6
  Add9/1 -> Build 3x3 Matrix/7
  Add3/1 -> Build 3x3 Matrix/8
  Gain/1 -> Add7/1, Add4/1
  Gain1/1 -> Add7/2, Add4/2
  Gain2/1 -> Add9/1, Add6/1
  Gain3/1 -> Add9/2, Add6/2
  Gain5/1 -> Add3/1, Add8/1
  Gain4/1 -> Add3/2, Add8/2
  Build 3x3 Matrix1/1 -> "M2 "/1
  q1^2-q2^2-q3^2+q4^2/1(Out1) -> Build 3x3 Matrix1/1
  Add11/1 -> Build 3x3 Matrix1/2
  Add5/1 -> Build 3x3 Matrix1/3
  Add14/1 -> Build 3x3 Matrix1/4
  Add15/1 -> Build 3x3 Matrix1/8
  -q1^2+q2^2-q3^2+q4^2/1(Out1) -> Build 3x3 Matrix1/5
  Add13/1 -> Build 3x3 Matrix1/7
  Add12/1 -> Build 3x3 Matrix1/6
  -q1^2-q2^2+q3^2+q4^2/1(Out1) -> Build 3x3 Matrix1/9
  q/1 -> Subsystem/1(q), -q1^2+q2^2-q3^2+q4^2/1(q), -q1^2-q2^2+q3^2+q4^2/1(q), q1^2-q2^2-q3^2+q4^2/1(q)
  Subsystem/1(2q1q2) -> Add11/1, Add14/1
  Subsystem/2(2q1q3) -> Add5/1, Add13/1
  Subsystem/3(2q1q4) -> Add15/2, Add12/2
  Subsystem/6(2q3q4) -> Add11/2, Add14/2
  Subsystem/5(2q2q4) -> Add13/2, Add5/2
  Subsystem/4(2q2q3) -> Add15/1, Add12/1

== system librarySimulink/Quaternions /Normalization  ==
  "q " : Inport
  4D-Norm : $bdroot/4D-Norm  SystemSampleTime=-1  VariantActivationTime=update diagram  Latency=0  AutoFrameSizeCalculation=off
  Divide : Product  Inputs=*/
  qNormalized : Outport
  wires:
  "q "/1 -> 4D-Norm/1, Divide/1
  4D-Norm/1 -> Divide/2
  Divide/1 -> qNormalized/1

== system librarySimulink/SRP torque/For Iterator Subsystem ==
  S_B : Inport
  Add : Sum
  Constant : Constant  Value=SRP.areas  VectorParams1D=off
  Constant1 : Constant  Value=SRP.positions  VectorParams1D=off
  Constant2 : Constant  Value=SRP.normalVects  VectorParams1D=off
  Constant3 : Constant  Value=SRP.rhoSValues  VectorParams1D=off
  Constant4 : Constant  Value=SRP.rhoDValues  VectorParams1D=off
  For Iterator : ForIterator  IterationLimit=SRP.nSurfaces
  Memory : Memory  InheritSampleTime=on
  Selector : Selector  InputPortWidth=SRP.nSurfaces  IndexOptions=Index vector (port)  Indices=[1 3]  OutputSizes=1
  Selector1 : Selector  NumberOfDimensions=2  InputPortWidth=[3,nSurfaces]  IndexOptions=Index vector (dialog),Index vector (port)  Indices=[1 2 3],[1 2 3]  OutputSizes=1,1
  Selector2 : Selector  NumberOfDimensions=2  InputPortWidth=3  IndexOptions=Index vector (dialog),Index vector (port)  Indices=[1 2 3],1  OutputSizes=1,1
  Selector3 : Selector  InputPortWidth=SRP.nSurfaces  IndexOptions=Index vector (port)  Indices=[1 3]  OutputSizes=1
  Selector4 : Selector  InputPortWidth=SRP.nSurfaces  IndexOptions=Index vector (port)  Indices=[1 3]  OutputSizes=1
  i-th torque : Subsystem
  T : Outport
  wires:
  Constant/1 -> Selector/1
  Constant1/1 -> Selector1/1
  Selector/1 -> i-th torque/1(area)
  Selector1/1 -> i-th torque/2(r)
  Constant2/1 -> Selector2/1
  Selector2/1 -> i-th torque/3(N_B)
  S_B/1 -> i-th torque/4(S_B)
  i-th torque/1(T) -> Add/1
  Memory/1 -> Add/2
  Add/1 -> Memory/1, T/1
  Constant3/1 -> Selector3/1
  Selector3/1 -> i-th torque/5(rhoS)
  Constant4/1 -> Selector4/1
  For Iterator/1 -> Selector/2, Selector1/2, Selector2/2, Selector3/2, Selector4/2
  Selector4/1 -> i-th torque/6(rhoD)

== system librarySimulink/Single Axis Rotation Matrix/If Action Subsystem ==
  angle : Inport
  Action Port : ActionPort  ActionPortLabel=if(u1 == 1)
  Build 3x3 Matrix : $bdroot/Build 3x3 Matrix  SystemSampleTime=-1  VariantActivationTime=update diagram  Latency=0  AutoFrameSizeCalculation=off
  Constant : Constant  Value=0
  Constant1 : Constant
  Cos : Trigonometry  Operator=cos
  Gain : Gain  Gain=-1
  Sin : Trigonometry
  A : Outport
  wires:
  Build 3x3 Matrix/1 -> A/1
  angle/1 -> Cos/1, Sin/1
  Constant1/1 -> Build 3x3 Matrix/1
  Constant/1 -> Build 3x3 Matrix/7, Build 3x3 Matrix/3, Build 3x3 Matrix/2, Build 3x3 Matrix/4
  Cos/1 -> Build 3x3 Matrix/9, Build 3x3 Matrix/5
  Gain/1 -> Build 3x3 Matrix/6
  Sin/1 -> Gain/1, Build 3x3 Matrix/8

== system librarySimulink/Single Axis Rotation Matrix/If Action Subsystem1 ==
  angle : Inport
  Action Port : ActionPort
  Build 3x3 Matrix : $bdroot/Build 3x3 Matrix  SystemSampleTime=-1  VariantActivationTime=update diagram  Latency=0  AutoFrameSizeCalculation=off
  Constant : Constant  Value=0
  Constant1 : Constant
  Cos : Trigonometry  Operator=cos
  Gain : Gain  Gain=-1
  Sin : Trigonometry
  A : Outport
  wires:
  angle/1 -> Sin/1, Cos/1
  Build 3x3 Matrix/1 -> A/1
  Cos/1 -> Build 3x3 Matrix/9, Build 3x3 Matrix/1
  Constant/1 -> Build 3x3 Matrix/8, Build 3x3 Matrix/6, Build 3x3 Matrix/2, Build 3x3 Matrix/4
  Sin/1 -> Gain/1, Build 3x3 Matrix/3
  Constant1/1 -> Build 3x3 Matrix/5
  Gain/1 -> Build 3x3 Matrix/7

== system librarySimulink/Single Axis Rotation Matrix/If Action Subsystem2 ==
  angle : Inport
  Action Port : ActionPort
  Build 3x3 Matrix : $bdroot/Build 3x3 Matrix  SystemSampleTime=-1  VariantActivationTime=update diagram  Latency=0  AutoFrameSizeCalculation=off
  Constant : Constant  Value=0
  Constant1 : Constant
  Cos : Trigonometry  Operator=cos
  Gain : Gain  Gain=-1
  Sin : Trigonometry
  A : Outport
  wires:
  angle/1 -> Sin/1, Cos/1
  Build 3x3 Matrix/1 -> A/1
  Constant/1 -> Build 3x3 Matrix/3, Build 3x3 Matrix/8, Build 3x3 Matrix/7, Build 3x3 Matrix/6
  Constant1/1 -> Build 3x3 Matrix/9
  Gain/1 -> Build 3x3 Matrix/2
  Sin/1 -> Build 3x3 Matrix/4, Gain/1
  Cos/1 -> Build 3x3 Matrix/5, Build 3x3 Matrix/1

== system librarySimulink/Spacecraft + Dual Spin/Dual Spin ==
  Mr : Inport
  Gain : Gain  Gain=1/spacecraft.dualSpin.Ir
  Integrator : Integrator  InitialCondition=1/spacecraft.dualSpin.wr0
  wr : Outport
  wr_dot : Outport  Port=2
  wires:
  Mr/1 -> Gain/1
  Gain/1 -> wr_dot/1, Integrator/1  "wr_dot"
  Integrator/1 -> wr/1  "wr"

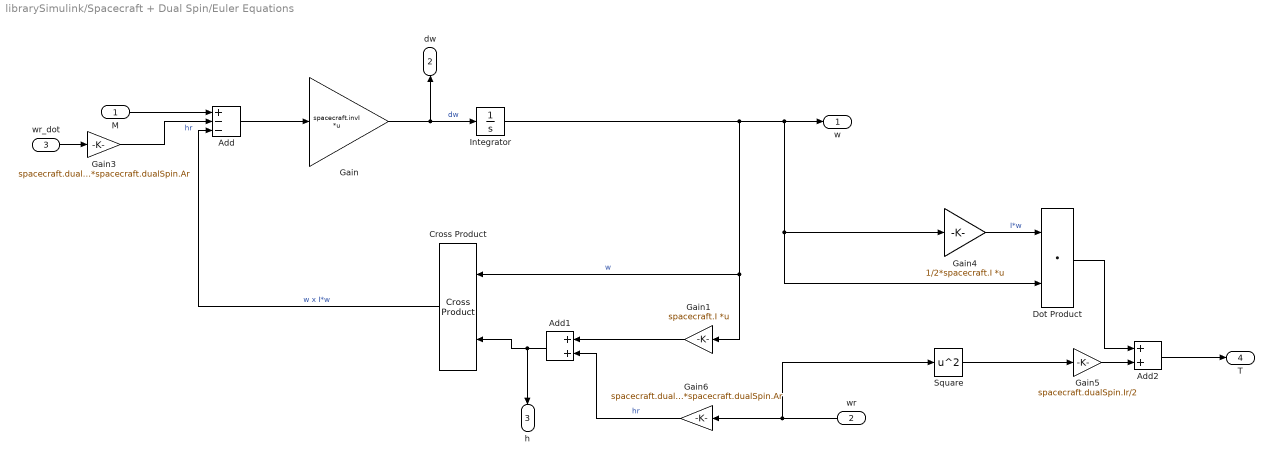
== system librarySimulink/Spacecraft + Dual Spin/Euler Equations ==
  M : Inport
  wr : Inport  Port=2
  "wr_dot " : Inport  Port=3
  Add : Sum  Inputs=+--
  Add1 : Sum
  Add2 : Sum
  Cross Product : $bdroot/Cross Product  SystemSampleTime=-1  VariantActivationTime=update diagram  Latency=0  AutoFrameSizeCalculation=off
  Dot Product : DotProduct  InputSameDT=on  OutDataTypeStr=Inherit: Inherit via internal rule
  Gain : Gain  Gain=spacecraft.invI  Multiplication=Matrix(K*u) (u vector)
  Gain1 : Gain  Gain=spacecraft.I  Multiplication=Matrix(K*u) (u vector)
  Gain3 : Gain  Gain=spacecraft.dualSpin.Ir*spacecraft.dualSpin.Ar
  Gain4 : Gain  Gain=1/2*spacecraft.I  Multiplication=Matrix(K*u) (u vector)
  Gain5 : Gain  Gain=spacecraft.dualSpin.Ir/2
  Gain6 : Gain  Gain=spacecraft.dualSpin.Ir*spacecraft.dualSpin.Ar
  Integrator : Integrator  InitialCondition=spacecraft.w0
  Square : Math  Operator=square  SaturateOnIntegerOverflow=on
  w : Outport
  dw : Outport  Port=2
  h : Outport  Port=3
  T : Outport  Port=4
  wires:
  Add/1 -> Gain/1
  M/1 -> Add/1
  Cross Product/1 -> Add/3  "w x I*w"
  Gain1/1 -> Add1/1
  Gain/1 -> Integrator/1, dw/1  "dw"
  wr/1 -> Gain6/1, Square/1
  Gain6/1 -> Add1/2  "hr"
  Add1/1 -> h/1, Cross Product/2
  "wr_dot "/1 -> Gain3/1
  Gain3/1 -> Add/2  "hr"
  Gain4/1 -> Dot Product/1  "I*w"
  Integrator/1 -> Cross Product/1, Gain1/1, w/1, Dot Product/2, Gain4/1  "w"
  Dot Product/1 -> Add2/1
  Gain5/1 -> Add2/2
  Square/1 -> Gain5/1
  Add2/1 -> T/1

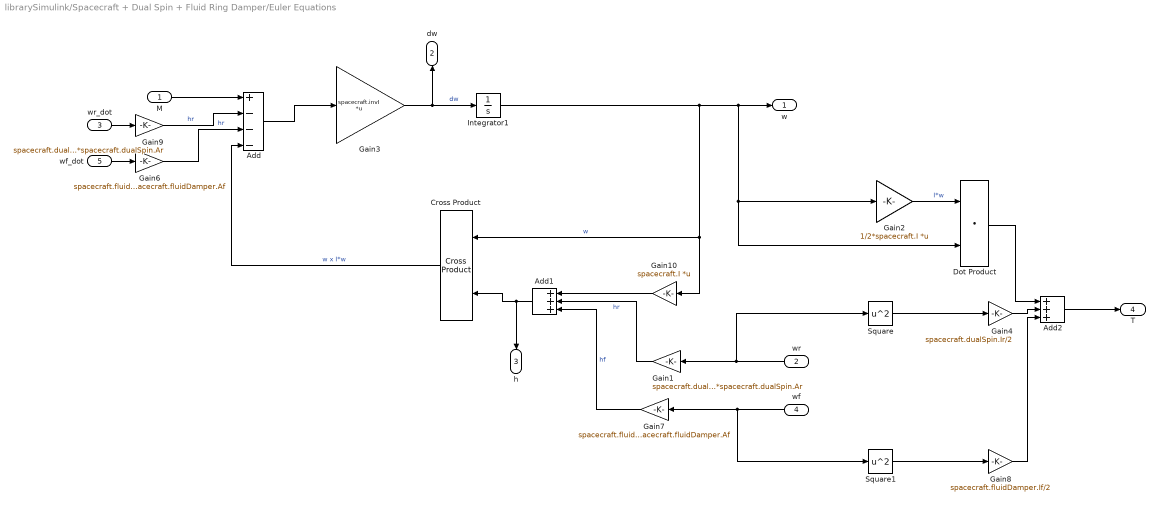
== system librarySimulink/Spacecraft + Dual Spin + Fluid Ring Damper/Euler Equations ==
  M : Inport
  wr : Inport  Port=2
  "wr_dot " : Inport  Port=3
  wf : Inport  Port=4
  wf_dot : Inport  Port=5
  Add : Sum  Inputs=+---
  Add1 : Sum  Inputs=+++
  Add2 : Sum  Inputs=+++
  Cross Product : $bdroot/Cross Product  SystemSampleTime=-1  VariantActivationTime=update diagram  Latency=0  AutoFrameSizeCalculation=off
  Dot Product : DotProduct  InputSameDT=on  OutDataTypeStr=Inherit: Inherit via internal rule
  Gain1 : Gain  Gain=spacecraft.dualSpin.Ir*spacecraft.dualSpin.Ar
  Gain10 : Gain  Gain=spacecraft.I  Multiplication=Matrix(K*u) (u vector)
  Gain2 : Gain  Gain=1/2*spacecraft.I  Multiplication=Matrix(K*u) (u vector)
  Gain3 : Gain  Gain=spacecraft.invI  Multiplication=Matrix(K*u) (u vector)
  Gain4 : Gain  Gain=spacecraft.dualSpin.Ir/2
  Gain6 : Gain  Gain=spacecraft.fluidDamper.If*spacecraft.fluidDamper.Af
  Gain7 : Gain  Gain=spacecraft.fluidDamper.If*spacecraft.fluidDamper.Af
  Gain8 : Gain  Gain=spacecraft.fluidDamper.If/2
  Gain9 : Gain  Gain=spacecraft.dualSpin.Ir*spacecraft.dualSpin.Ar
  Integrator1 : Integrator  InitialCondition=spacecraft.w0
  Square : Math  Operator=square  SaturateOnIntegerOverflow=on
  Square1 : Math  Operator=square  SaturateOnIntegerOverflow=on
  w : Outport
  dw : Outport  Port=2
  h : Outport  Port=3
  T : Outport  Port=4
  wires:
  Add/1 -> Gain3/1
  M/1 -> Add/1
  Cross Product/1 -> Add/4  "w x I*w"
  Gain10/1 -> Add1/1
  Gain3/1 -> Integrator1/1, dw/1  "dw"
  wr/1 -> Gain1/1, Square/1
  Gain1/1 -> Add1/2  "hr"
  Add1/1 -> h/1, Cross Product/2
  "wr_dot "/1 -> Gain9/1
  Gain9/1 -> Add/2  "hr"
  Gain2/1 -> Dot Product/1  "I*w"
  Integrator1/1 -> Gain10/1, Cross Product/1, w/1, Gain2/1, Dot Product/2  "w"
  Dot Product/1 -> Add2/1
  Square/1 -> Gain4/1
  Add2/1 -> T/1
  wf_dot/1 -> Gain6/1
  Gain6/1 -> Add/3  "hr"
  wf/1 -> Square1/1, Gain7/1
  Gain7/1 -> Add1/3  "hf"
  Square1/1 -> Gain8/1
  Gain8/1 -> Add2/3
  Gain4/1 -> Add2/2

== system librarySimulink/Spacecraft + Dual Spin + Fluid Ring Damper/Fluid Ring Damper ==
  note: Use c*(w_x + w_f) to simulate
      | a control action. Use c*(w_f - w_x)
      | to simulate a viscous effect.
  w : Inport
  Add : Sum
  Constant : Constant  Value=spacecraft.fluidDamper.Af  VectorParams1D=off
  Dot Product : DotProduct  InputSameDT=on  OutDataTypeStr=Inherit: Inherit via internal rule
  Gain : Gain  Gain=-spacecraft.fluidDamper.c/spacecraft.fluidDamper.If
  Integrator : Integrator  InitialCondition=spacecraft.fluidDamper.wf0
  wf : Outport
  wf_dot : Outport  Port=2
  wires:
  w/1 -> Dot Product/1
  Constant/1 -> Dot Product/2
  Add/1 -> Gain/1
  Gain/1 -> wf_dot/1, Integrator/1  "wf_dot"
  Integrator/1 -> wf/1, Add/2  "wf"
  Dot Product/1 -> Add/1

== system librarySimulink/Magnetic Torque/Subsystem/R^3*H0//r^3 ==
  rNorm : Inport
  Constant : Constant  Value=3
  Constant1 : Constant  Value=3
  Divide : Product  Inputs=**/
  H0 : Constant  Value=((-29615e-9)^2 + (-1728e-9)^2 + 5186e-9^2)^(1/2)
  Power : Math  Operator=pow  SaturateOnIntegerOverflow=on
  Power1 : Math  Operator=pow  SaturateOnIntegerOverflow=on
  R_EARTH : Constant  Value=R_EARTH
  Out1 : Outport
  wires:
  H0/1 -> Divide/2
  Power/1 -> Divide/1
  Power1/1 -> Divide/3
  Divide/1 -> Out1/1
  Constant1/1 -> Power1/2
  rNorm/1 -> Power1/1
  Constant/1 -> Power/2
  R_EARTH/1 -> Power/1

== system librarySimulink/Quaternions /M2/-q1^2+q2^2-q3^2+q4^2 ==
  q : Inport
  Add : Sum  Inputs=-+-+
  Demux : Demux
  Square{,1..3} (4 alike) : Math  Operator=square  SaturateOnIntegerOverflow=on
  Out1 : Outport
  wires:
  q/1 -> Demux/1
  Demux/1 -> Square/1
  Demux/2 -> Square1/1
  Demux/3 -> Square2/1
  Demux/4 -> Square3/1
  Add/1 -> Out1/1
  Square/1 -> Add/1
  Square1/1 -> Add/2
  Square2/1 -> Add/3
  Square3/1 -> Add/4

== system librarySimulink/Quaternions /M2/-q1^2-q2^2+q3^2+q4^2 ==
  q : Inport
  Add : Sum  Inputs=--++
  Demux : Demux
  Square{,1..3} (4 alike) : Math  Operator=square  SaturateOnIntegerOverflow=on
  Out1 : Outport
  wires:
  q/1 -> Demux/1
  Demux/1 -> Square/1
  Demux/2 -> Square1/1
  Demux/3 -> Square2/1
  Demux/4 -> Square3/1
  Add/1 -> Out1/1
  Square/1 -> Add/1
  Square1/1 -> Add/2
  Square2/1 -> Add/3
  Square3/1 -> Add/4

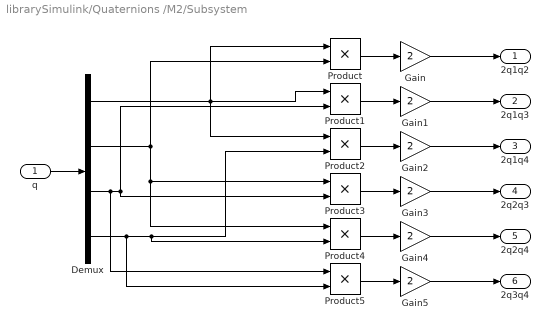
== system librarySimulink/Quaternions /M2/Subsystem ==
  q : Inport
  Demux : Demux
  Gain{,1..5} (6 alike) : Gain  Gain=2
  Product{,1..5} (6 alike) : Product
  2q1q2 : Outport
  2q1q3 : Outport  Port=2
  2q1q4 : Outport  Port=3
  2q2q3 : Outport  Port=4
  2q2q4 : Outport  Port=5
  2q3q4 : Outport  Port=6
  wires:
  q/1 -> Demux/1
  Demux/1 -> Product2/1, Product1/1, Product/1
  Demux/2 -> Product4/1, Product3/1, Product/2
  Demux/3 -> Product5/1, Product3/2, Product1/2
  Demux/4 -> Product5/2, Product4/2, Product2/2
  Product/1 -> Gain/1
  Product1/1 -> Gain1/1
  Product3/1 -> Gain3/1
  Product2/1 -> Gain2/1
  Product5/1 -> Gain5/1
  Product4/1 -> Gain4/1
  Gain/1 -> 2q1q2/1
  Gain1/1 -> 2q1q3/1
  Gain2/1 -> 2q1q4/1
  Gain3/1 -> 2q2q3/1
  Gain5/1 -> 2q3q4/1
  Gain4/1 -> 2q2q4/1

== system librarySimulink/Quaternions /M2/q1^2-q2^2-q3^2+q4^2 ==
  q : Inport
  Add : Sum  Inputs=+--+
  Demux : Demux
  Square{,1..3} (4 alike) : Math  Operator=square  SaturateOnIntegerOverflow=on
  Out1 : Outport
  wires:
  q/1 -> Demux/1
  Demux/1 -> Square/1
  Demux/2 -> Square1/1
  Demux/3 -> Square2/1
  Demux/4 -> Square3/1
  Add/1 -> Out1/1
  Square/1 -> Add/1
  Square1/1 -> Add/2
  Square2/1 -> Add/3
  Square3/1 -> Add/4

== system librarySimulink/Quaternions /M2/qi*qj  ==
  q : Inport
  Demux1 : Demux
  Product{,1..5} (6 alike) : Product
  q1q2 : Outport
  q3q4 : Outport  Port=2
  q1q3 : Outport  Port=3
  q2q4 : Outport  Port=4
  q1q4 : Outport  Port=5
  q2q3 : Outport  Port=6
  wires:
  Demux1/3 -> Product2/2, Product3/2, Product1/1
  Product2/1 -> q2q3/1  "q2q3"
  Product4/1 -> q2q4/1  "q2q4"
  Demux1/1 -> Product5/1, Product3/1, Product/1
  Demux1/2 -> Product4/1, Product2/1, Product/2
  Demux1/4 -> Product5/2, Product4/2, Product1/2
  Product5/1 -> q1q4/1  "q1q4"
  Product/1 -> q1q2/1  "q1q2"
  Product3/1 -> q1q3/1  "q1q3"
  Product1/1 -> q3q4/1  "q34"
  q/1 -> Demux1/1

== system librarySimulink/SRP torque/For Iterator Subsystem/i-th torque ==
  area : Inport
  r : Inport  Port=2
  N_B : Inport  Port=3
  S_B : Inport  Port=4
  rhoS : Inport  Port=5
  rhoD : Inport  Port=6
  Dot Product : DotProduct  InputSameDT=on  OutDataTypeStr=Inherit: Inherit via internal rule
  If : If
  If Action Subsystem : Subsystem  TreatAsAtomicUnit=on
  If Action Subsystem1 : Subsystem  TreatAsAtomicUnit=on
  Merge : Merge
  N_B1 : InportShadow  Port=3
  S_B1 : InportShadow  Port=4
  T : Outport
  wires:
  N_B/1 -> Dot Product/1
  S_B/1 -> Dot Product/2
  Dot Product/1 -> If/1
  Merge/1 -> T/1
  If/2 -> If Action Subsystem/Action
  If Action Subsystem/1(T) -> Merge/2
  If/1 -> If Action Subsystem1/Action
  If Action Subsystem1/1(T) -> Merge/1
  area/1 -> If Action Subsystem1/1(area)
  N_B1/1 -> If Action Subsystem1/2(N_B)
  S_B1/1 -> If Action Subsystem1/3(S_B)
  r/1 -> If Action Subsystem1/4(r)
  rhoD/1 -> If Action Subsystem1/6(rhoD)
  rhoS/1 -> If Action Subsystem1/5(rhoS)

== system librarySimulink/SRP torque/For Iterator Subsystem/i-th torque/If Action Subsystem ==
  Action Port : ActionPort
  Constant : Constant  Value=0
  Mux : Mux  Inputs=3
  T : Outport
  wires:
  Mux/1 -> T/1
  Constant/1 -> Mux/2, Mux/1, Mux/3

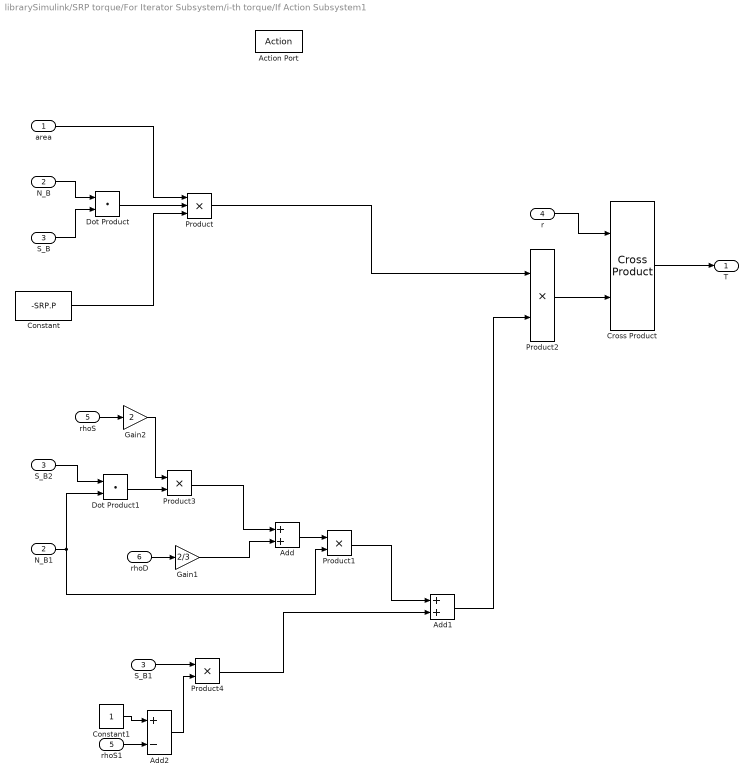
== system librarySimulink/SRP torque/For Iterator Subsystem/i-th torque/If Action Subsystem1 ==
  area : Inport
  N_B : Inport  Port=2
  S_B : Inport  Port=3
  r : Inport  Port=4
  rhoS : Inport  Port=5
  rhoD : Inport  Port=6
  Action Port : ActionPort
  Add : Sum
  Add1 : Sum
  Add2 : Sum  Inputs=+-
  Constant : Constant  Value=-SRP.P
  Constant1 : Constant
  Cross Product : $bdroot/Cross Product  SystemSampleTime=-1  VariantActivationTime=update diagram  Latency=0  AutoFrameSizeCalculation=off
  Dot Product : DotProduct  InputSameDT=on  OutDataTypeStr=Inherit: Inherit via internal rule
  Dot Product1 : DotProduct  InputSameDT=on  OutDataTypeStr=Inherit: Inherit via internal rule
  Gain1 : Gain  Gain=2/3
  Gain2 : Gain  Gain=2
  N_B1 : InportShadow  Port=2
  Product : Product  Inputs=3
  Product{1..4} (4 alike) : Product
  S_B1 : InportShadow  Port=3
  S_B2 : InportShadow  Port=3
  rhoS1 : InportShadow  Port=5
  T : Outport
  wires:
  N_B/1 -> Dot Product/1
  S_B/1 -> Dot Product/2
  area/1 -> Product/1
  Dot Product/1 -> Product/2
  Constant/1 -> Product/3
  S_B1/1 -> Product4/1
  S_B2/1 -> Dot Product1/1
  N_B1/1 -> Product1/2, Dot Product1/2
  Dot Product1/1 -> Product3/2
  Product3/1 -> Add/1
  Gain1/1 -> Add/2
  Add/1 -> Product1/1
  Product1/1 -> Add1/1
  Product4/1 -> Add1/2
  Product/1 -> Product2/1
  Add1/1 -> Product2/2
  Cross Product/1 -> T/1
  r/1 -> Cross Product/1
  Product2/1 -> Cross Product/2
  rhoS/1 -> Gain2/1
  Gain2/1 -> Product3/1
  rhoD/1 -> Gain1/1
  rhoS1/1 -> Add2/2
  Constant1/1 -> Add2/1
  Add2/1 -> Product4/2

== matlab function librarySimulink/Magnetic Torque (MATLAB function)/MATLAB Function ==
  data: t input; r input; M output; A_BN input; m input
function M = fcn(t, r, A_BN, m)

g10 = -29615e-9; g11 = -1728e-9; h11 = 5186e-9;
H0 = sqrt(g10^2 + g11^2 + h11^2);

R_EARTH = 6378;
N_EARTH = 2*pi/(165*365*24*3600);
rNorm = norm(r);
rVers = r/rNorm;

mVers = [sind(11.5)*cos(N_EARTH*t); sind(11.5)*sin(N_EARTH*t);  cosd(11.5)];

b_N = R_EARTH^3*H0/rNorm^3*(3*dot(mVers,rVers)*rVers - mVers);

b_B = A_BN*b_N;

M = cross(m,b_B);

== matlab function librarySimulink/SRP torque (MATLAB function)/MATLAB Function ==
  data: S_B input; M output; areaValues input; positions input; normalVects input; rhoSValues input; rhoDValues input
function M = fcn(S_B,areaValues,positions,normalVects,rhoSValues,rhoDValues)
P = 1358/3e8;
M = [0;0;0];
for i=1:length(areaValues)
    area = areaValues(i);
    r = positions(:,i);
    N_B = normalVects(:,i);
    rhoS = rhoSValues(i); rhoD = rhoDValues(i);
    
    if dot(N_B,S_B) > 0
        F = -P*area*dot(N_B,S_B)*(...
            (1-rhoS)*S_B + (2*rhoS*dot(S_B,N_B) + 2/3*rhoD)*N_B);
        M = M + cross(r,F);
    else
        M = M + [0;0;0];
    end
end
